simulink model "matlab_control_demo_model_basic"  (R2022b)
settings: Solver=FixedStepAuto  StartTime=0.0  StopTime=inf  RelTol=1e-3
libraries: simulink x1
settings Model: Creator=v-zbraude  LastModifiedBy=edufford

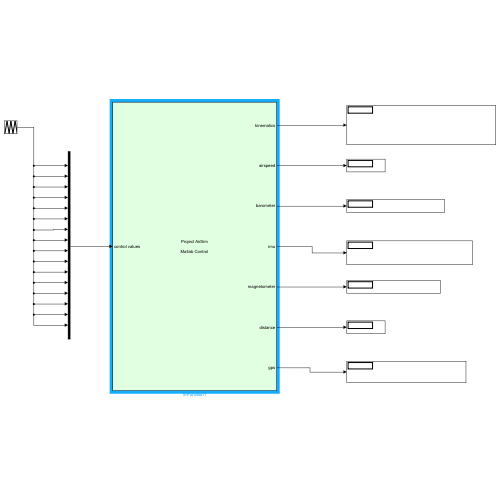
[thumbnail: Simulink's stored preview of the top-level diagram]
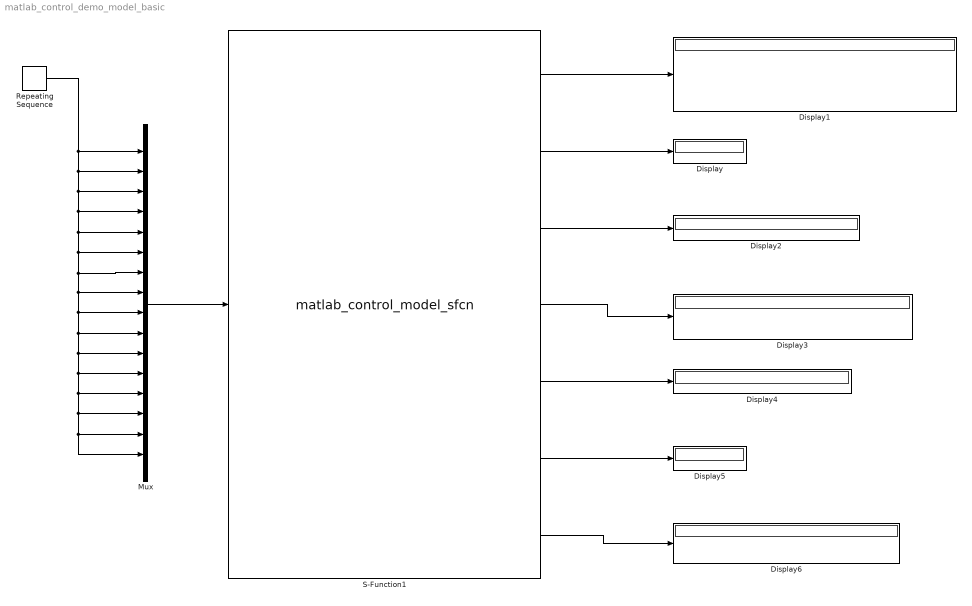
== system matlab_control_demo_model_basic ==
  Display{,1..6} (7 alike) : Display
  Mux : Mux  Inputs=16
  Repeating Sequence : simulink/Sources/Repeating Sequence  rep_seq_t=[0 5 10]  rep_seq_y=[0 1 0]
  S-Function1 : S-Function  Priority=20  FunctionName=matlab_control_model_sfcn  Parameters=hostname,portnumber,timestep  SFunctionDeploymentMode=off  EnableBusSupport=off  mask{hostname=*, portnumber=8998, timestep=0.003}
      mask prompts: hostname "Host name:"; portnumber "Port number:"; timestep "AirSim time step:"
      mask Display:
      | disp("Project AirSim\n\n")
      | disp("\n\nMatlab Control")
      | port_label('input',1,'control values')
      | port_label('output',1,'kinematics')
      | port_label('output',2,'airspeed')
      | port_label('output',3,'barometer')
      | port_label('output',4,'imu')
      | port_label('output',5,'magnetometer')
      | port_label('output',6,'distance')
      | port_label('output',7,'gps')
  wires:
  S-Function1/1 -> Display1/1
  S-Function1/7 -> Display6/1
  S-Function1/6 -> Display5/1
  S-Function1/5 -> Display4/1
  S-Function1/4 -> Display3/1
  S-Function1/3 -> Display2/1
  S-Function1/2 -> Display/1
  Repeating Sequence/1 -> Mux/1, Mux/2, Mux/3, Mux/7, Mux/8, Mux/9, Mux/10, Mux/11, Mux/14, Mux/15, Mux/16, Mux/13, Mux/12, Mux/6, Mux/5, Mux/4
  Mux/1 -> S-Function1/1
